simulink model "main_program"  (R2025b)
settings: Solver=VariableStepAuto  StartTime=0.0  StopTime=10.0  RelTol=1e-3
InitFcn:
  | initial_param;
undefined symbols (not defined in the file or in its folder): control, Control, SystemDynamics, Vehicle
libraries: slpidlib x1
settings Model: Creator=tomer  LastModifiedBy=tomer

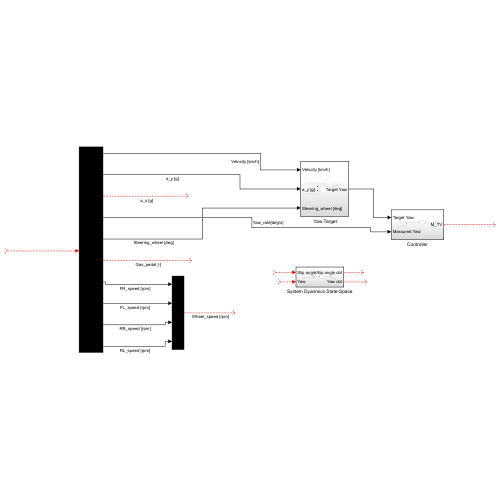
[thumbnail: Simulink's stored preview of the top-level diagram]
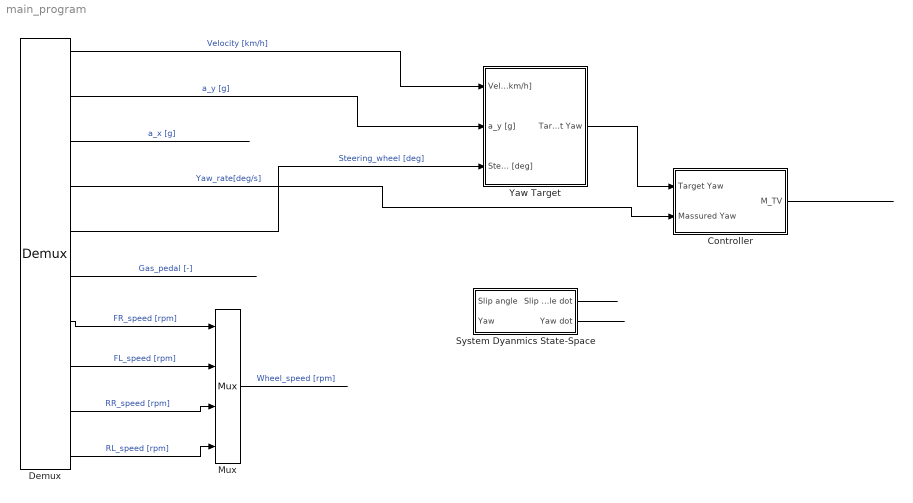
== system main_program ==
  " Yaw Target" : Subsystem
  Controller : Subsystem
  Demux : Demux  Outputs=10
  Mux : Mux
  System Dyanmics State-Space : Subsystem
  wires:
  Demux/1 -> " Yaw Target"/1(Velocity [km/h])  "Velocity [km/h]"
  Demux/2 -> " Yaw Target"/2(a_y [g])  "a_y [g]"
  Demux/3 -> ?  "a_x [g]"
  Demux/4 -> Controller/2(Massured Yaw)  "Yaw_rate[deg/s]"
  Demux/5 -> " Yaw Target"/3(Steering_wheel [deg])  "Steering_wheel [deg]"
  Demux/6 -> ?  "Gas_pedal [-]"
  Demux/7 -> Mux/1  "FR_speed [rpm]"
  Demux/8 -> Mux/2  "FL_speed [rpm]"
  Demux/9 -> Mux/3  "RR_speed [rpm]"
  Demux/10 -> Mux/4  "RL_speed [rpm]"
  Mux/1 -> ?  "Wheel_speed [rpm]"
  ? -> Demux/1
  " Yaw Target"/1(Target Yaw) -> Controller/1(Target Yaw)
  Controller/1(M_TV) -> ?
  ? -> System Dyanmics State-Space/1(Slip angle)
  ? -> System Dyanmics State-Space/2(Yaw)
  System Dyanmics State-Space/1(Slip angle dot) -> ?
  System Dyanmics State-Space/2(Yaw dot) -> ?

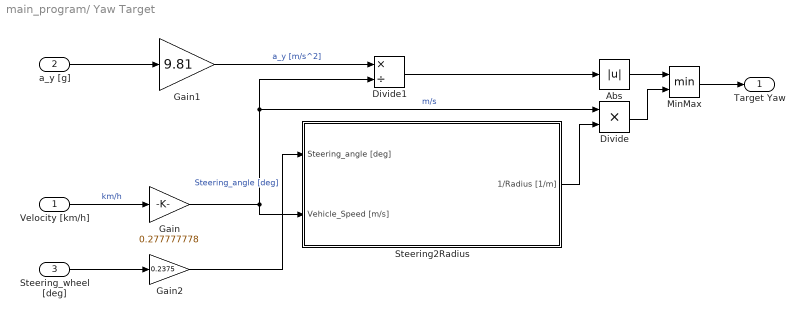
== system main_program/ Yaw Target ==
  Velocity [km/h] : Inport
  a_y [g] : Inport  Port=2
  Steering_wheel [deg] : Inport  Port=3
  Abs : Abs  SaturateOnIntegerOverflow=off
  Divide : Product  Inputs=**
  Divide1 : Product  Inputs=*/
  Gain : Gain  Gain=0.277777778
  Gain1 : Gain  Gain=9.81
  Gain2 : Gain  Gain=0.2375
  MinMax : MinMax  Inputs=2
  Steering2Radius : Subsystem
  Target Yaw : Outport
  wires:
  a_y [g]/1 -> Gain1/1
  Velocity [km/h]/1 -> Gain/1  "km/h"
  Steering_wheel [deg]/1 -> Gain2/1
  Steering2Radius/1(1/Radius [1/m]) -> Divide/2
  Gain2/1 -> Steering2Radius/1(Steering_angle [deg])  "Steering_angle [deg]"
  Gain/1 -> Steering2Radius/2(Vehicle_Speed [m/s]), Divide/1, Divide1/2  "m/s"
  Gain1/1 -> Divide1/1  "a_y [m/s^2]"
  Divide1/1 -> Abs/1
  Abs/1 -> MinMax/1
  Divide/1 -> MinMax/2
  MinMax/1 -> Target Yaw/1

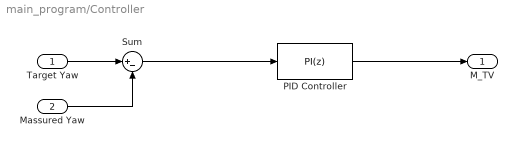
== system main_program/Controller ==
  Target Yaw : Inport
  Massured Yaw : Inport  Port=2
  PID Controller : slpidlib/PID Controller  Controller=PI  Form=Parallel  TimeDomain=Discrete-time  UseExternalTs=off  SampleTime=control.Ts  IntegratorMethod=Forward Euler  FilterMethod=Forward Euler  ControllerParametersSource=internal  P=control.Kp  I=control.Ki  UseKiTs=off  D=0  UseExternalDerivativeSource=off  N=100  UseFilter=on  TunerSelectOption=Transfer Function Based (PID Tuner App)  InitialConditionSource=internal  InitialConditionForIntegrator=0  InitialConditionForFilter=0  DifferentiatorICPrevScaledInput=0  ExternalReset=none  TrackingMode=off  Kt=1  LimitOutput=on  SatLimitsSource=internal  UpperSaturationLimit=Control.MaxYawMoment  LowerSaturationLimit=-Control.MaxYawMoment  LinearizeAsGain=on  AntiWindupMode=clamping  Kb=1  LimitIntegrator=off  UpperIntegratorSaturationLimit=inf  LowerIntegratorSaturationLimit=-inf  POutMin=[]  POutMax=[]  IOutMin=[]  IOutMax=[]  DOutMin=[]  DOutMax=[]  NOutMin=[]  NOutMax=[]  SumOutMin=[]  SumOutMax=[]  SaturationOutMin=[]  SaturationOutMax=[]  PParamMin=[]  PParamMax=[]  IParamMin=[]  IParamMax=[]  DParamMin=[]  DParamMax=[]  NParamMin=[]  NParamMax=[]  KbParamMin=[]  KbParamMax=[]  KtParamMin=[]  KtParamMax=[]  KbOutMin=[]  KbOutMax=[]  KtOutMin=[]  KtOutMax=[]  IntegratorOutMin=[]  IntegratorOutMax=[]  FilterOutMin=[]  FilterOutMax=[]  SumI1OutMin=[]  SumI1OutMax=[]  SumI2OutMin=[]  SumI2OutMax=[]  SumI3OutMin=[]  SumI3OutMax=[]  SumI4OutMin=[]  SumI4OutMax=[]  SumDOutMin=[]  SumDOutMax=[]  DifferentiatorOutMin=[]  DifferentiatorOutMax=[]  FilterDiffOutCoefMin=[]  FilterDiffOutCoefMax=[]  ReciprocalOutMin=[]  ReciprocalOutMax=[]  SumDenOutMin=[]  SumDenOutMax=[]  SumNumOutMin=[]  SumNumOutMax=[]  DivideOutMin=[]  DivideOutMax=[]  UdiffTsProdOutMin=[]  UdiffTsProdOutMax=[]  NTsProdOutMin=[]  NTsProdOutMax=[]  UintegralTsProdOutMin=[]  UintegralTsProdOutMax=[]  UngainTsProdOutMin=[]  UngainTsProdOutMax=[]  ClampingZeroOutDataTypeStr=Inherit: Inherit via back propagation  ClampingZeroOutMin=[]  ClampingZeroOutMax=[]  FilterDenConstantOutDataTypeStr=Inherit: Inherit via back propagation  FilterDenConstantOutMin=[]  FilterDenConstantOutMax=[]  PCopyOutDataTypeStr=Inherit: Inherit via back propagation  PCopyOutMin=[]  PCopyOutMax=[]  NCopyOutDataTypeStr=Inherit: Inherit via back propagation  NCopyOutMin=[]  NCopyOutMax=[]  IntegratorContinuousStateAttributes=''  IntegratorStateMustResolveToSignalObject=off  IntegratorRTWStateStorageClass=Auto  FilterContinuousStateAttributes=''  FilterStateMustResolveToSignalObject=off  FilterRTWStateStorageClass=Auto  ParallelPVariant=InternalParameters  IdealPVariant=Disabled  IVariant=InternalParameters  DVariant=Disabled  IntegratorVariant=Discrete  SatVariant=Enabled  AWVariant=DiscClampingParallel  PCopyVariant=Disabled  TRVariant=Disabled  FdbkBlocksVariant=Forward  IdealPFdbkVariant=Disabled  SatFdbkVariant=Disabled  DerivativeFilterVariant=Disabled  NVariant=Disabled  NCopyVariant=Disabled_SignalSpec  FilterICVariant=Disabled  IntegratorICVariant=InternalICs  ExternalResetVariant=Disabled  TRSumVariant=Passthrough  SumFdbkVariant=Disabled  SumVariant=Sum_PI  TsampFilterVariant=InternalTs  TsampNgainVariant=Passthrough  TsampIntegralVariant=Disabled_SignalSpec  ExternalSaturationOutDataTypeStr=Inherit: Same as second input  DerivativeSourceVariant=Disabled  PreIntVariant=InternalPreInt
  Sum : Sum  Inputs=|+-
  M_TV : Outport
  wires:
  Target Yaw/1 -> Sum/1
  Massured Yaw/1 -> Sum/2
  Sum/1 -> PID Controller/1
  PID Controller/1 -> M_TV/1

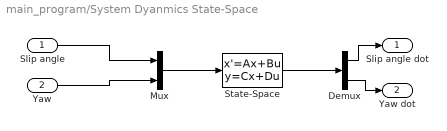
== system main_program/System Dyanmics State-Space ==
  Slip angle : Inport
  Yaw : Inport  Port=2
  Demux : Demux  Outputs=2
  Mux : Mux  Inputs=2
  State-Space : StateSpace  A=SystemDynamics.A  B=SystemDynamics.B  C=zeros(2)  D=zeros(2)  InitialCondition=0
  Slip angle dot : Outport
  Yaw dot : Outport  Port=2
  wires:
  Yaw/1 -> Mux/2
  Slip angle/1 -> Mux/1
  Mux/1 -> State-Space/1
  State-Space/1 -> Demux/1
  Demux/1 -> Slip angle dot/1
  Demux/2 -> Yaw dot/1

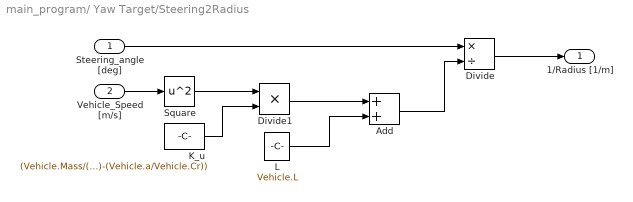
== system main_program/ Yaw Target/Steering2Radius ==
  Steering_angle [deg] : Inport
  Vehicle_Speed [m/s] : Inport  Port=2
  Add : Sum
  Divide : Product  Inputs=*/
  Divide1 : Product  Inputs=**
  K_u : Constant  Value=(Vehicle.Mass/(Vehicle.a+Vehicle.b))*((Vehicle.b/Vehicle.Cf)-(Vehicle.a/Vehicle.Cr))
  L : Constant  Value=Vehicle.L
  Square : Math  Operator=square
  1/Radius [1/m] : Outport
  wires:
  Steering_angle [deg]/1 -> Divide/1
  Vehicle_Speed [m/s]/1 -> Square/1
  Square/1 -> Divide1/1
  K_u/1 -> Divide1/2
  Divide1/1 -> Add/1
  Add/1 -> Divide/2
  L/1 -> Add/2
  Divide/1 -> 1/Radius [1/m]/1
